simulink model "VCU_EnergyMgnt"  (R2023b)
settings: Solver=FixedStepAuto  StartTime=0.0  StopTime=0.1  FixedStep=0.01  RelTol=1e-3
undefined symbols (not defined in the file or in its folder): DiscIntNeverNeededParam
libraries: simulink x10
settings Model: Creator=Administrator  LastModifiedBy=Administrator
settings OptimizationCC: DefaultParameterBehavior=Inlined  EnhancedBackFolding=on  PassReuseOutputArgsAs=Individual arguments  ZeroExternalMemoryAtStartup=off  ZeroInternalMemoryAtStartup=off  OptimizeBlockOrder=speed  DifferentSizesBufferReuse=on  OptimizationCustomize=off  EfficientTunableParamExpr=on
settings DebuggingCC: ParameterTunabilityLossMsg=error
settings HardwareCC: ProdBitPerPointer=32  ProdBitPerSizeT=32  ProdBitPerPtrDiffT=32  ProdLargestAtomicInteger=Long  ProdLargestAtomicFloat=Double  ProdWordSize=32  ProdHWDeviceType=ARM Compatible->ARM Cortex-M
settings SFSimCC: MATLABDynamicMemAlloc=off
settings RTWCC: Description=Embedded Coder  SystemTargetFile=ert.tlc  GenCodeOnly=on  TemplateMakefile=ert_default_tmf  GenerateReport=on  IncludeHyperlinkInReport=on  LaunchReport=on  GenerateTraceInfo=on  GenerateTraceReport=on  GenerateCodeReplacementReport=on
settings CodeAppCC: ForceParamTrailComments=on  IgnoreCustomStorageClasses=off  OperatorAnnotations=on  SimulinkDataObjDesc=on  SFDataObjDesc=on  InsertBlockDesc=on
settings ERTTargetCC: TargetLangStandard=C99 (ISO)  GenerateSampleERTMain=on  InlinedParameterPlacement=NonHierarchical  ERTCustomFileTemplate=example_file_process.tlc

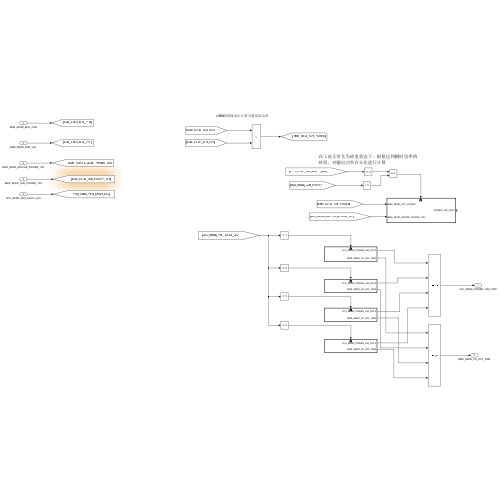
[thumbnail: Simulink's stored preview of the top-level diagram]
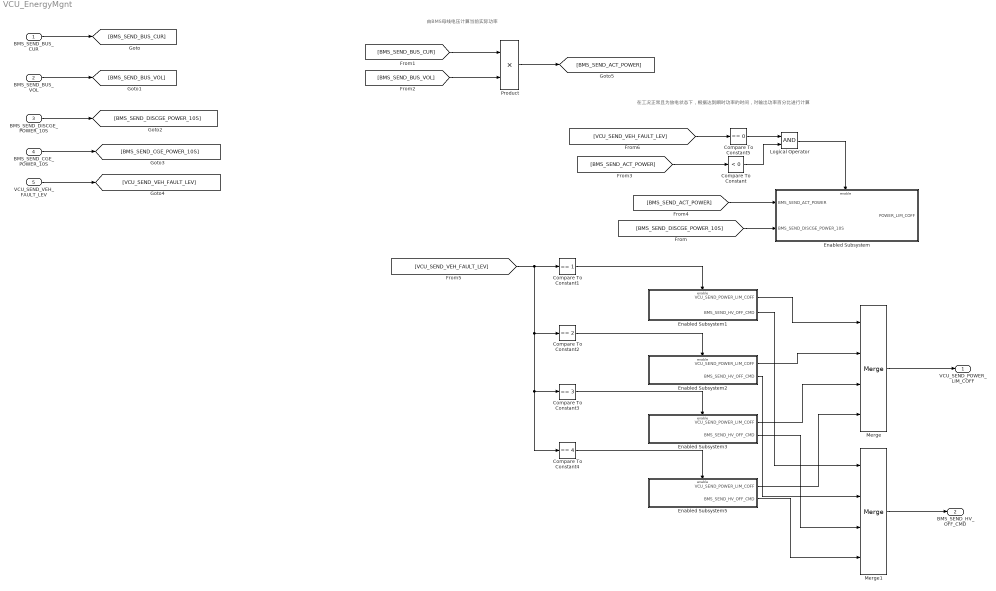
== system VCU_EnergyMgnt ==
  note: 在工况正常且为放电状态下，根据达到瞬时功率的时间，对输出功率百分比进行计算
  note: 由BMS母线电压计算当前实际功率
  BMS_SEND_BUS_CUR : Inport
  BMS_SEND_BUS_VOL : Inport  Port=2
  BMS_SEND_DISCGE_POWER_10S : Inport  Port=3
  BMS_SEND_CGE_POWER_10S : Inport  Port=4
  VCU_SEND_VEH_FAULT_LEV : Inport  Port=5
  Compare To Constant : simulink/Logic and Bit Operations/Compare To Constant  relop=<  const=0  OutDataTypeStr=boolean
  Compare To Constant1 : simulink/Logic and Bit Operations/Compare To Constant  relop===  const=1  OutDataTypeStr=boolean
  Compare To Constant2 : simulink/Logic and Bit Operations/Compare To Constant  relop===  const=2  OutDataTypeStr=boolean
  Compare To Constant3 : simulink/Logic and Bit Operations/Compare To Constant  relop===  const=3  OutDataTypeStr=boolean
  Compare To Constant4 : simulink/Logic and Bit Operations/Compare To Constant  relop===  const=4  OutDataTypeStr=boolean
  Compare To Constant5 : simulink/Logic and Bit Operations/Compare To Constant  relop===  const=0  OutDataTypeStr=boolean
  Enabled Subsystem : Subsystem  TreatAsAtomicUnit=on
  Enabled Subsystem1 : Subsystem  TreatAsAtomicUnit=on
  Enabled Subsystem2 : Subsystem  TreatAsAtomicUnit=on
  Enabled Subsystem3 : Subsystem  TreatAsAtomicUnit=on
  Enabled Subsystem5 : Subsystem  TreatAsAtomicUnit=on
  Logical Operator : Logic  AllPortsSameDT=off  OutDataTypeStr=boolean
  Merge : Merge  Inputs=4
  Merge1 : Merge  Inputs=4
  Product : Product  OutDataTypeStr=single
  VCU_SEND_POWER_LIM_COFF : Outport
  BMS_SEND_HV_OFF_CMD : Outport  Port=2
  wires:
  BMS_SEND_BUS_CUR/1 -> [BMS_SEND_BUS_CUR]
  BMS_SEND_BUS_VOL/1 -> [BMS_SEND_BUS_VOL]
  BMS_SEND_DISCGE_POWER_10S/1 -> [BMS_SEND_DISCGE_POWER_10S]
  BMS_SEND_CGE_POWER_10S/1 -> [BMS_SEND_CGE_POWER_10S]
  VCU_SEND_VEH_FAULT_LEV/1 -> [VCU_SEND_VEH_FAULT_LEV]
  [BMS_SEND_BUS_CUR] -> Product/1
  [BMS_SEND_BUS_VOL] -> Product/2
  Product/1 -> [BMS_SEND_ACT_POWER]
  [BMS_SEND_ACT_POWER] -> Compare To Constant/1
  [BMS_SEND_ACT_POWER] -> Enabled Subsystem/1(BMS_SEND_ACT_POWER)
  [BMS_SEND_DISCGE_POWER_10S] -> Enabled Subsystem/2(BMS_SEND_DISCGE_POWER_10S)
  [VCU_SEND_VEH_FAULT_LEV] -> Compare To Constant4/1, Compare To Constant3/1, Compare To Constant2/1, Compare To Constant1/1
  Compare To Constant1/1 -> Enabled Subsystem1/Enable
  Compare To Constant2/1 -> Enabled Subsystem2/Enable
  Compare To Constant3/1 -> Enabled Subsystem3/Enable
  Compare To Constant4/1 -> Enabled Subsystem5/Enable
  Enabled Subsystem1/1(VCU_SEND_POWER_LIM_COFF) -> Merge/1
  Enabled Subsystem2/1(VCU_SEND_POWER_LIM_COFF) -> Merge/2
  Enabled Subsystem3/1(VCU_SEND_POWER_LIM_COFF) -> Merge/3
  Enabled Subsystem5/1(VCU_SEND_POWER_LIM_COFF) -> Merge/4
  Enabled Subsystem1/2(BMS_SEND_HV_OFF_CMD) -> Merge1/1
  Enabled Subsystem2/2(BMS_SEND_HV_OFF_CMD) -> Merge1/2
  Enabled Subsystem3/2(BMS_SEND_HV_OFF_CMD) -> Merge1/3
  Enabled Subsystem5/2(BMS_SEND_HV_OFF_CMD) -> Merge1/4
  Merge/1 -> VCU_SEND_POWER_LIM_COFF/1
  Merge1/1 -> BMS_SEND_HV_OFF_CMD/1
  [VCU_SEND_VEH_FAULT_LEV] -> Compare To Constant5/1
  Compare To Constant5/1 -> Logical Operator/1
  Compare To Constant/1 -> Logical Operator/2
  Logical Operator/1 -> Enabled Subsystem/Enable

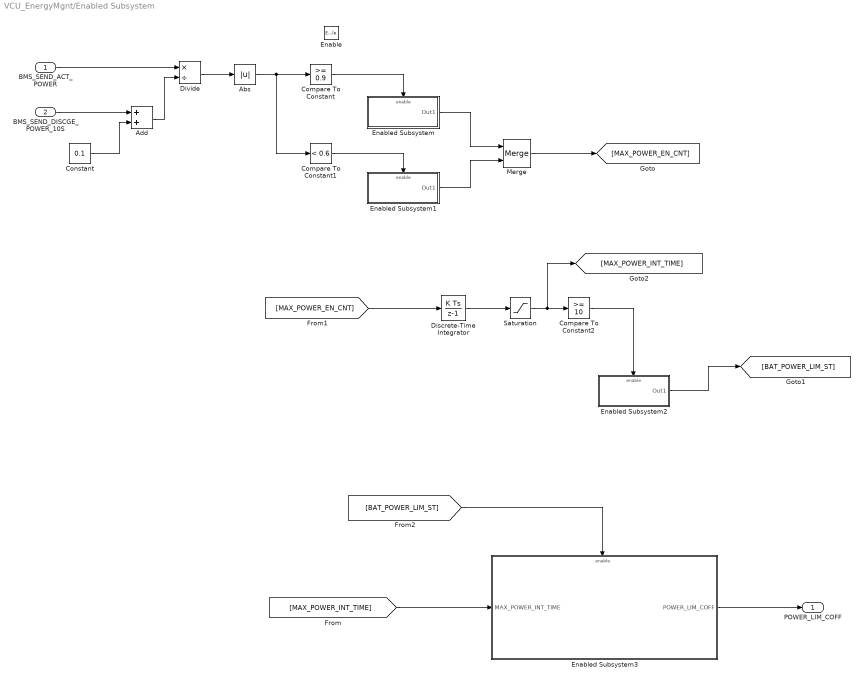
== system VCU_EnergyMgnt/Enabled Subsystem ==
  BMS_SEND_ACT_POWER : Inport
  BMS_SEND_DISCGE_POWER_10S : Inport  Port=2
  Enable : EnablePort
  Abs : Abs  SaturateOnIntegerOverflow=off
  Add : Sum
  Compare To Constant : simulink/Logic and Bit Operations/Compare To Constant  relop=>=  const=0.9  OutDataTypeStr=boolean
  Compare To Constant1 : simulink/Logic and Bit Operations/Compare To Constant  relop=<  const=0.6  OutDataTypeStr=boolean
  Compare To Constant2 : simulink/Logic and Bit Operations/Compare To Constant  relop=>=  const=10  OutDataTypeStr=boolean
  Constant : Constant  Value=0.1
  Discrete-Time Integrator : DiscreteIntegrator  SampleTime=-1  ICPrevOutput=DiscIntNeverNeededParam  ICPrevScaledInput=DiscIntNeverNeededParam
  Divide : Product  Inputs=*/  RndMeth=Zero  SaturateOnIntegerOverflow=on
  Enabled Subsystem : Subsystem  TreatAsAtomicUnit=on
  Enabled Subsystem1 : Subsystem  TreatAsAtomicUnit=on
  Enabled Subsystem2 : Subsystem  TreatAsAtomicUnit=on
  Enabled Subsystem3 : Subsystem  TreatAsAtomicUnit=on
  Merge : Merge
  Saturation : Saturate  UpperLimit=1500  LowerLimit=-1500
  POWER_LIM_COFF : Outport
  wires:
  BMS_SEND_DISCGE_POWER_10S/1 -> Add/1
  Constant/1 -> Add/2
  BMS_SEND_ACT_POWER/1 -> Divide/1
  Add/1 -> Divide/2
  Divide/1 -> Abs/1
  Abs/1 -> Compare To Constant1/1, Compare To Constant/1
  Compare To Constant/1 -> Enabled Subsystem/Enable
  Compare To Constant1/1 -> Enabled Subsystem1/Enable
  Enabled Subsystem/1(Out1) -> Merge/1
  Enabled Subsystem1/1(Out1) -> Merge/2
  Merge/1 -> [MAX_POWER_EN_CNT]
  [MAX_POWER_EN_CNT] -> Discrete-Time Integrator/1
  Discrete-Time Integrator/1 -> Saturation/1
  Saturation/1 -> [MAX_POWER_INT_TIME], Compare To Constant2/1
  Compare To Constant2/1 -> Enabled Subsystem2/Enable
  Enabled Subsystem2/1(Out1) -> [BAT_POWER_LIM_ST]
  [BAT_POWER_LIM_ST] -> Enabled Subsystem3/Enable
  [MAX_POWER_INT_TIME] -> Enabled Subsystem3/1(MAX_POWER_INT_TIME)
  Enabled Subsystem3/1(POWER_LIM_COFF) -> POWER_LIM_COFF/1

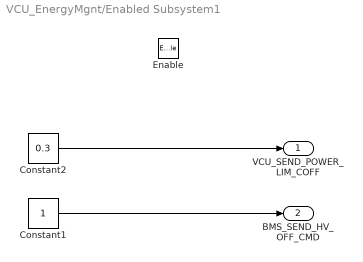
== system VCU_EnergyMgnt/Enabled Subsystem1 ==
  Enable : EnablePort
  Constant1 : Constant
  Constant2 : Constant  Value=0.3
  VCU_SEND_POWER_LIM_COFF : Outport
  BMS_SEND_HV_OFF_CMD : Outport  Port=2
  wires:
  Constant1/1 -> BMS_SEND_HV_OFF_CMD/1
  Constant2/1 -> VCU_SEND_POWER_LIM_COFF/1

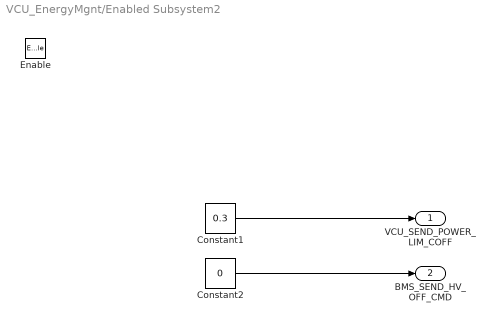
== system VCU_EnergyMgnt/Enabled Subsystem2 ==
  Enable : EnablePort
  Constant1 : Constant  Value=0.3
  Constant2 : Constant  Value=0
  VCU_SEND_POWER_LIM_COFF : Outport
  BMS_SEND_HV_OFF_CMD : Outport  Port=2
  wires:
  Constant1/1 -> VCU_SEND_POWER_LIM_COFF/1
  Constant2/1 -> BMS_SEND_HV_OFF_CMD/1

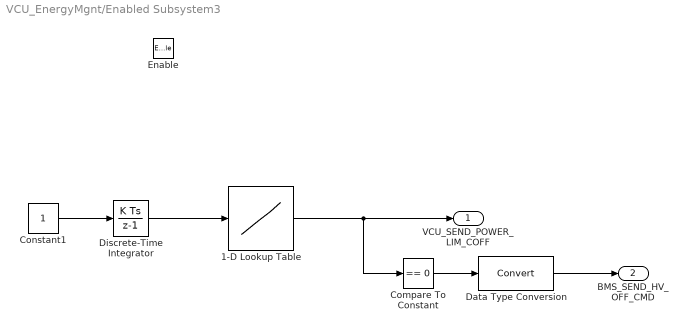
== system VCU_EnergyMgnt/Enabled Subsystem3 ==
  Enable : EnablePort
  1-D Lookup Table : Lookup_n-D  NumberOfTableDimensions=1  BreakpointsForDimension1=[0 500 1000]  Table=[0.1 0.1 0]  InternalRulePriority=Speed  RndMeth=Simplest
  Compare To Constant : simulink/Logic and Bit Operations/Compare To Constant  relop===  const=0  OutDataTypeStr=boolean
  Constant1 : Constant
  Data Type Conversion : DataTypeConversion  SaturateOnIntegerOverflow=off  RndMeth=Floor
  Discrete-Time Integrator : DiscreteIntegrator  SampleTime=-1  ICPrevOutput=DiscIntNeverNeededParam  ICPrevScaledInput=DiscIntNeverNeededParam
  VCU_SEND_POWER_LIM_COFF : Outport
  BMS_SEND_HV_OFF_CMD : Outport  Port=2
  wires:
  Constant1/1 -> Discrete-Time Integrator/1
  1-D Lookup Table/1 -> Compare To Constant/1, VCU_SEND_POWER_LIM_COFF/1
  Discrete-Time Integrator/1 -> 1-D Lookup Table/1
  Compare To Constant/1 -> Data Type Conversion/1
  Data Type Conversion/1 -> BMS_SEND_HV_OFF_CMD/1

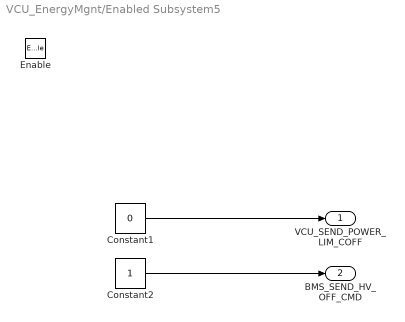
== system VCU_EnergyMgnt/Enabled Subsystem5 ==
  Enable : EnablePort
  Constant1 : Constant  Value=0
  Constant2 : Constant
  VCU_SEND_POWER_LIM_COFF : Outport
  BMS_SEND_HV_OFF_CMD : Outport  Port=2
  wires:
  Constant2/1 -> BMS_SEND_HV_OFF_CMD/1
  Constant1/1 -> VCU_SEND_POWER_LIM_COFF/1

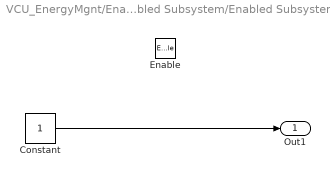
== system VCU_EnergyMgnt/Enabled Subsystem/Enabled Subsystem ==
  Enable : EnablePort
  Constant : Constant  OutDataTypeStr=single
  Out1 : Outport
  wires:
  Constant/1 -> Out1/1

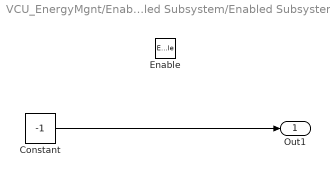
== system VCU_EnergyMgnt/Enabled Subsystem/Enabled Subsystem1 ==
  Enable : EnablePort
  Constant : Constant  Value=-1  OutDataTypeStr=single
  Out1 : Outport
  wires:
  Constant/1 -> Out1/1

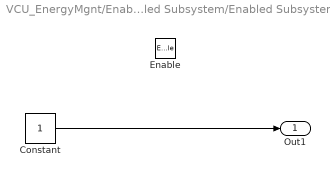
== system VCU_EnergyMgnt/Enabled Subsystem/Enabled Subsystem2 ==
  Enable : EnablePort
  Constant : Constant  OutDataTypeStr=single
  Out1 : Outport
  wires:
  Constant/1 -> Out1/1

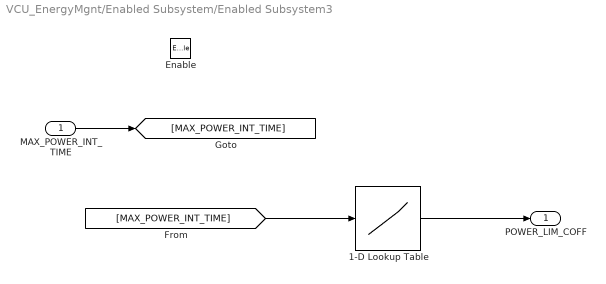
== system VCU_EnergyMgnt/Enabled Subsystem/Enabled Subsystem3 ==
  MAX_POWER_INT_TIME : Inport
  Enable : EnablePort
  1-D Lookup Table : Lookup_n-D  NumberOfTableDimensions=1  BreakpointsForDimension1=[0 10 15]  Table=[1 1 0.5]  InternalRulePriority=Speed  RndMeth=Simplest
  POWER_LIM_COFF : Outport
  wires:
  MAX_POWER_INT_TIME/1 -> [MAX_POWER_INT_TIME]
  [MAX_POWER_INT_TIME] -> 1-D Lookup Table/1
  1-D Lookup Table/1 -> POWER_LIM_COFF/1
